simulink model "LQG_Dead_Zone_1"  (R2018a)
settings: Solver=ode45  StartTime=0.0  StopTime=500  RelTol=1e-6  EnableMultiTasking=on
values from neighbouring files (symbols this model uses):
  A = stateSpaceModel.A    [System_Control.m]    (also in script2.m)
  B = stateSpaceModel.B    [System_Control.m]    (also in script2.m)
  C = stateSpaceModel.C    [System_Control.m]    (also in script2.m)
  Nbar = Nu+K*Nx    [System_Control.m]    (also in script2.m)
  Ts = stateSpaceModel.Ts    [System_Control.m]    (also in script2.m)
undefined symbols (not defined in the file or in its folder): Atrue, Btrue, Ctrue, DiscIntNeverNeededParam, Dtrue, K, M
libraries: simulink x2
settings Model: Creator=jomle  LastModifiedBy=Pedro
settings DataIOCC: LimitDataPoints=on  SaveFormat=Array
settings OptimizationCC: LifeSpan=inf
settings DebuggingCC: SFUnexpectedBacktrackingDiag=warning  SFNoUnconditionalDefaultTransitionDiag=warning  SFExecutionAtInitializationDiag=none
settings HardwareCC: ProdBitPerPointer=32  ProdBitPerSizeT=32  ProdBitPerPtrDiffT=32  ProdLargestAtomicFloat=None  ProdIntDivRoundTo=Undefined  ProdEndianess=Unspecified  ProdWordSize=32  ProdHWDeviceType=32-bit Generic
settings ModelReferenceCC: PropagateSignalLabelsOutOfModel=off
settings CodeAppCC: StateflowObjectComments=on
settings GRTTargetCC: TargetLangStandard=C89/C90 (ANSI)
settings ConfigComp: CovMetricSettings=dw  CovHtmlReporting=on  CovSaveCumulativeToWorkspaceVar=on  CovSaveSingleToWorkspaceVar=on  CovExternalEMLEnable=off

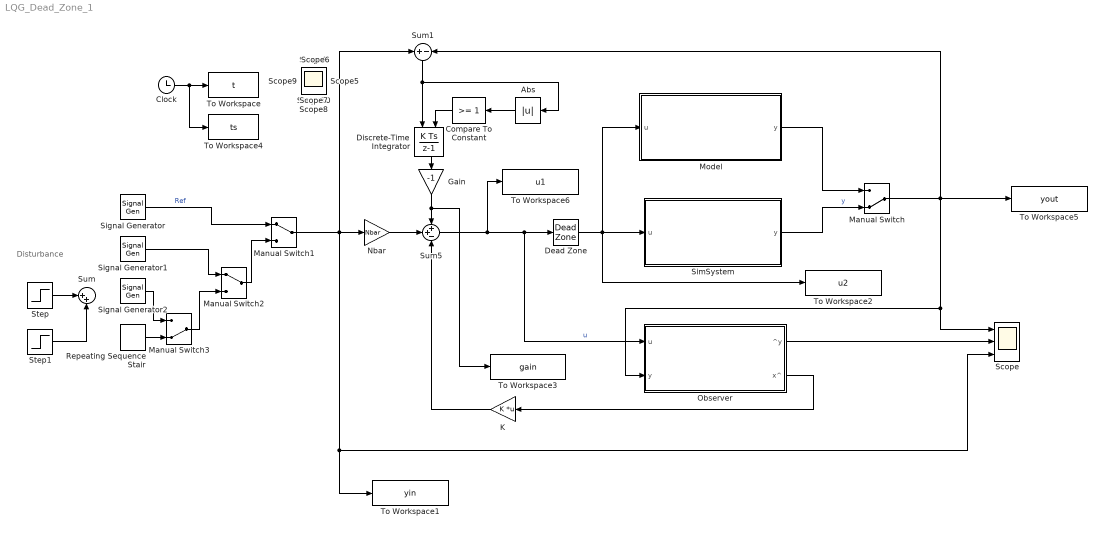
== system LQG_Dead_Zone_1 ==
  note: Disturbance
  Abs : Abs
  Clock : Clock
  Compare To Constant : simulink/Logic and Bit Operations/Compare To Constant  relop=>=  const=1  OutDataTypeStr=boolean
  Dead Zone : DeadZone  LowerValue=-0.1  UpperValue=0.1  SaturateOnIntegerOverflow=on
  Discrete-Time Integrator : DiscreteIntegrator  gainval=20e-3  ExternalReset=sampled level  SampleTime=-1  ICPrevOutput=DiscIntNeverNeededParam  ICPrevScaledInput=DiscIntNeverNeededParam
  Gain : Gain  Gain=-1
  K : Gain  Gain=K  Multiplication=Matrix(K*u)
  Manual Switch : ManualSwitch  CurrentSetting=0
  Manual Switch1 : ManualSwitch
  Manual Switch2 : ManualSwitch
  Manual Switch3 : ManualSwitch  CurrentSetting=0
  Model : Subsystem
  Nbar : Gain  Gain=Nbar
  Observer : Subsystem  Tag=Observer  Description=Observer
  Repeating Sequence Stair : simulink/Sources/Repeating Sequence Stair  OutValues=[1 4 2 3].'  tsamp=10  OutMin=[]  OutMax=[]  OutDataTypeStr=double  OutputDataTypeScalingMode=double  OutDataType=fixdt(0,8)  ConRadixGroup=Best Precision: Vector-wise  OutScaling=2^-12
  Scope : Scope  NumInputPorts=3
  Signal Generator : SignalGenerator  WaveForm=square  Amplitude=4  Frequency=1/50
  Signal Generator1 : SignalGenerator  WaveForm=sawtooth  Amplitude=4  Frequency=1/50
  Signal Generator2 : SignalGenerator  Amplitude=4  Frequency=1/50
  SimSystem : Subsystem
  Step : Step  Time=2  Before=-1  SampleTime=0.1
  Step1 : Step  Time=4  Before=1  After=-1  SampleTime=0.1
  Sum : Sum  Inputs=|++
  Sum1 : Sum  Inputs=+|-
  Sum5 : Sum  Inputs=++-
  To Workspace : ToWorkspace  VariableName=t  SampleTime=-1
  To Workspace1 : ToWorkspace  VariableName=yin  SaveFormat=Structure With Time  SampleTime=Ts
  To Workspace2 : ToWorkspace  VariableName=u2  SaveFormat=Structure With Time  SampleTime=Ts
  To Workspace3 : ToWorkspace  VariableName=gain  SaveFormat=Structure With Time  SampleTime=Ts
  To Workspace4 : ToWorkspace  VariableName=ts  SampleTime=Ts
  To Workspace5 : ToWorkspace  VariableName=yout  SaveFormat=Structure With Time  SampleTime=Ts
  To Workspace6 : ToWorkspace  VariableName=u1  SaveFormat=Structure With Time  SampleTime=Ts
  Scope{2..10} (9 alike) : Scope
  wires:
  Clock/1 -> To Workspace4/1, To Workspace/1
  Sum5/1 -> To Workspace6/1, Dead Zone/1, Observer/1(u)  "u"
  Step/1 -> Sum/1
  Step1/1 -> Sum/2
  Observer/1(^y) -> Scope/2
  Observer/2(x^) -> K/1
  Manual Switch/1 -> Scope/1, Observer/2(y), Sum1/2, To Workspace5/1
  Model/1(y) -> Manual Switch/1
  SimSystem/1(y) -> Manual Switch/2  "y"
  Dead Zone/1 -> To Workspace2/1, Model/1(u), SimSystem/1(u)
  Sum1/1 -> Discrete-Time Integrator/1, Abs/1
  Discrete-Time Integrator/1 -> Gain/1
  Nbar/1 -> Sum5/2
  K/1 -> Sum5/3
  Compare To Constant/1 -> Discrete-Time Integrator/2
  Abs/1 -> Compare To Constant/1
  Manual Switch1/1 -> Sum1/1, To Workspace1/1, Scope/3, Nbar/1
  Gain/1 -> To Workspace3/1, Sum5/1
  Signal Generator/1 -> Manual Switch1/1  "Ref"
  Signal Generator1/1 -> Manual Switch2/1
  Manual Switch2/1 -> Manual Switch1/2
  Repeating Sequence Stair/1 -> Manual Switch3/2
  Manual Switch3/1 -> Manual Switch2/2
  Signal Generator2/1 -> Manual Switch3/1

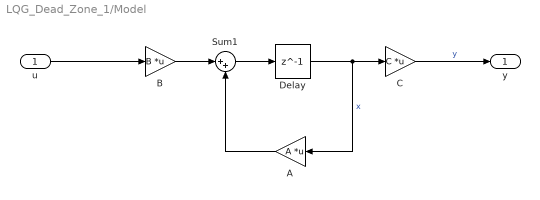
== system LQG_Dead_Zone_1/Model ==
  u : Inport
  "A " : Gain  Gain=A  Multiplication=Matrix(K*u)
  B : Gain  Gain=B  Multiplication=Matrix(K*u)
  C : Gain  Gain=C  Multiplication=Matrix(K*u)
  Delay : Delay  DelayLength=1  InitialCondition=0  SampleTime=Ts
  Sum1 : Sum  Inputs=|++
  y : Outport  VectorParamsAs1DForOutWhenUnconnected=on
  wires:
  u/1 -> B/1
  "A "/1 -> Sum1/2
  B/1 -> Sum1/1
  Delay/1 -> "A "/1, C/1  "x"
  Sum1/1 -> Delay/1
  C/1 -> y/1  "y"

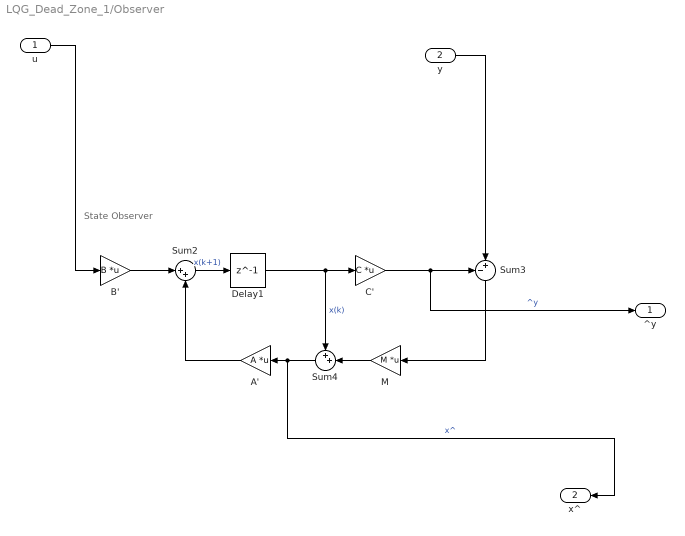
== system LQG_Dead_Zone_1/Observer ==
  note: State Observer
  u : Inport
  y : Inport  Port=2
  A' : Gain  Gain=A  Multiplication=Matrix(K*u)
  B' : Gain  Gain=B  Multiplication=Matrix(K*u)
  C' : Gain  Gain=C  Multiplication=Matrix(K*u)
  Delay1 : Delay  DelayLength=1  InitialCondition=0  SampleTime=Ts
  M : Gain  Gain=M  Multiplication=Matrix(K*u)
  Sum2 : Sum  Inputs=|++
  Sum3 : Sum  Inputs=-+|
  Sum4 : Sum  Inputs=++|
  ^y : Outport  VectorParamsAs1DForOutWhenUnconnected=on
  x^ : Outport  Port=2  VectorParamsAs1DForOutWhenUnconnected=on
  wires:
  M/1 -> Sum4/2
  Sum3/1 -> M/1
  Sum4/1 -> x^/1, A'/1  "x^"
  y/1 -> Sum3/2
  C'/1 -> ^y/1, Sum3/1  "^y"
  A'/1 -> Sum2/2
  Delay1/1 -> Sum4/1, C'/1  "x(k)"
  B'/1 -> Sum2/1
  Sum2/1 -> Delay1/1  "x(k+1)"
  u/1 -> B'/1

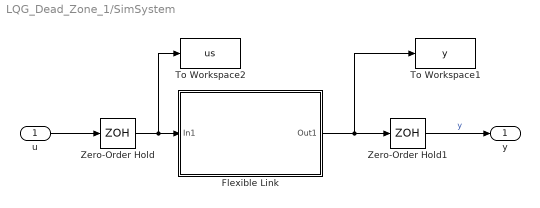
== system LQG_Dead_Zone_1/SimSystem ==
  u : Inport
  Flexible Link : Subsystem
      mask Display: image('quanserlink.jpg')
  To Workspace1 : ToWorkspace  VariableName=y  SampleTime=-1
  To Workspace2 : ToWorkspace  VariableName=us  SampleTime=Ts
  Zero-Order Hold : ZeroOrderHold  SampleTime=Ts
  Zero-Order Hold1 : ZeroOrderHold  SampleTime=Ts
  y : Outport  VectorParamsAs1DForOutWhenUnconnected=on
  wires:
  Flexible Link/1(Out1) -> To Workspace1/1, Zero-Order Hold1/1
  Zero-Order Hold/1 -> To Workspace2/1, Flexible Link/1(In1)
  Zero-Order Hold1/1 -> y/1  "y"
  u/1 -> Zero-Order Hold/1

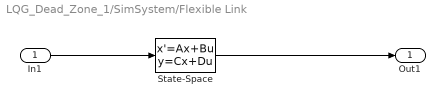
== system LQG_Dead_Zone_1/SimSystem/Flexible Link ==
  In1 : Inport
  State-Space : StateSpace  A=Atrue  B=Btrue  C=Ctrue  D=Dtrue  InitialCondition=0
  Out1 : Outport  VectorParamsAs1DForOutWhenUnconnected=on
  wires:
  State-Space/1 -> Out1/1
  In1/1 -> State-Space/1
